simulink model "linear_plunger_model"  (R2025a)
settings: Solver=VariableStepAuto  StartTime=0.0  StopTime=0.1  MaxStep=1e-6  RelTol=1e-3
InitFcn:
  | run param_file.m
values from neighbouring files (symbols this model uses):
  param = struct()    [Copy_of_param_file.m]    (also in param_file.m; param_file_loss_vs_freq.m; param_file_original.m; param_file_turbine.m)
settings Model: Creator=user  LastModifiedBy=user

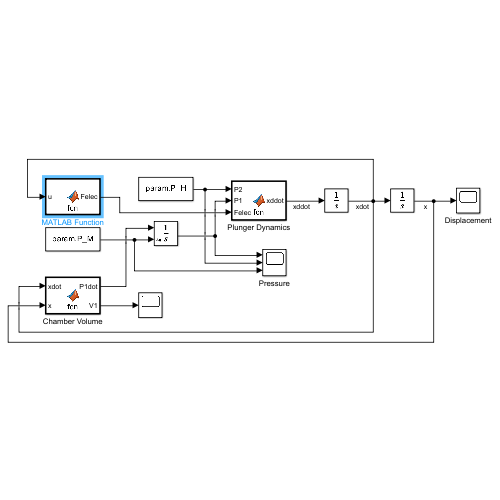
[thumbnail: Simulink's stored preview of the top-level diagram]
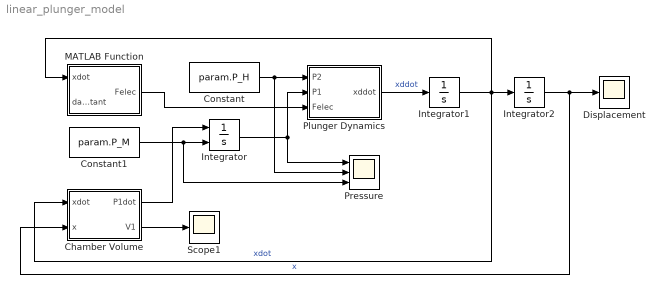
== system linear_plunger_model ==
  Chamber Volume : MATLAB Function  TreatAsAtomicUnit=on
  Constant : Constant  Value=param.P_H
  Constant1 : Constant  Value=param.P_M
  Displacement : Scope
      settings: ActiveDisplayYMinimum=-1  ActiveDisplayYMaximum=1
  Integrator : Integrator  InitialConditionSource=external  InitialCondition=param.P_initial
  Integrator1 : Integrator
  Integrator2 : Integrator
  MATLAB Function : MATLAB Function  TreatAsAtomicUnit=on
  Plunger Dynamics : MATLAB Function  TreatAsAtomicUnit=on
  Pressure : Scope  NumInputPorts=3
      settings: ActiveDisplayYMinimum=1.7210433908321168E+6  ActiveDisplayYMaximum=1.8980609482510954E+7  DataLoggingVariableName=ScopeData2
  Scope1 : Scope
      settings: ActiveDisplayYMinimum=-1  ActiveDisplayYMaximum=1
  wires:
  Chamber Volume/1(P1dot) -> Integrator/1
  Integrator/1 -> Plunger Dynamics/2(P1), Pressure/1
  Constant/1 -> Pressure/2, Plunger Dynamics/1(P2)
  Plunger Dynamics/1(xddot) -> Integrator1/1  "xddot"
  Integrator1/1 -> MATLAB Function/1(xdot), Chamber Volume/1(xdot), Integrator2/1  "xdot"
  Integrator2/1 -> Displacement/1, Chamber Volume/2(x)  "x"
  Chamber Volume/2(V1) -> Scope1/1
  Constant1/1 -> Integrator/2, Pressure/3
  MATLAB Function/1(Felec) -> Plunger Dynamics/3(Felec)

== matlab function linear_plunger_model/Plunger Dynamics ==
  data: P2 input; xddot output; P1 input; param parameter; Felec input
function xddot = fcn(P2, P1, param, Felec)

xddot = (1/param.plunger_mass) * (param.Aplunger*(P2-P1) - Felec);

== matlab function linear_plunger_model/Chamber Volume ==
  data: P1dot output; param parameter; xdot input; x input; V1 output
function [P1dot, V1] = fcn(param, xdot, x)

V1 = param.V1_0 - param.Aplunger*x;
P1dot = (param.beta/V1) * (param.Aplunger * xdot);

== matlab function linear_plunger_model/MATLAB Function ==
  data: xdot input; Felec output; damping_constant input
function Felec = fcn(xdot, damping_constant)

Felec = damping_constant * xdot;
